simulink library "Lib_Turbo_TurbinePSI_TMATS_org"  (Simulink 10.0)
settings: Solver=ode45  StartTime=0.0  StopTime=10.0  RelTol=1e-3  EnableMultiTasking=on
undefined symbols (not defined in the file): stripchar_TMATS
libraries: Lib_Solve_DataOut_TMATS x1
Description:
  | Thomas Modules
settings Model: Creator=jwchapm2  LastModifiedBy=bhisma

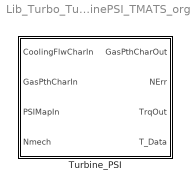
== system Lib_Turbo_TurbinePSI_TMATS_org ==
  Turbine_PSI : Subsystem  mask(T-MATS: Turbine_PSI Library Block){X_T_Map_PRpVec_M=[ 3.000  8.000], Y_T_Map_NcpVec_M=[60 80  110], T_T_Map_PSIArray_M=[0 0; 0 0; 0 0], X_T_Map_PRwVec_M=[ 3.000  8.000], Y_T_Map_NcwVec_M=[60 80  110], T_T_Map_WoWArray_M=[0 0;0 0; 0 0], s_T_hi_M=0.1, s_T_Nc_M=0.0243, s_T_Wc_M=0.4504, s_T_PR_M=0.9736, s_T_Eff_M=0.9984, CFlwEn_M=off, T_CoolFlwPos_M=0, gamma_M=1.4, Rt_M=0.1, iDesign_M=2, NcDes_M=100, EffDes_M=0.9328, PRDes_M=5, NDes_M=10000, FVar_M=strcat('iDes_',stripchar_TMATS(gcb),'.bin')}
      mask prompts: X_T_Map_PRpVec_M "X_T_Map_PRpVec_M - Turbine Map Pressure Ratio Vector (X-axis)(nx1)"; Y_T_Map_NcpVec_M "Y_T_Map_NcpVec_M - Turbine Map Corrected Speed Vector (Y-axis)(mx1)"; T_T_Map_PSIArray_M "T_T_Map_PSIArray_M - Turbine Map PSIMAPI Array (PSIMAPI = f(Nc,PR))(mxn)"; X_T_Map_PRwVec_M "X_T_Map_PRwVec_M - Turbine Map Pressure Ratio Vector (X-axis)(rx1)"; Y_T_Map_NcwVec_M "Y_T_Map_NcwVec_M - Turbine Map Corrected Speed Vector (Y-axis)(qx1)"; T_T_Map_WoWArray_M "T_T_Map_WoWArray_M - Turbine Map Flow Array (WoW=f(Nc,PR))(qxr)"; s_T_hi_M "s_T_hi_M - Corrected Entalpy Constant (T_hi)"; s_T_Nc_M "s_T_Nc_M - Corrected Speed Scalar Constant (T_Nc)"; s_T_Wc_M "s_T_Wc_M - Flow Scalar Constant (T_Wc)"; s_T_PR_M "s_T_PR_M - Pressure Ratio Scalar Constant (T_PR)"; s_T_Eff_M "s_T_Eff_M - Efficiency Scalar Constant (T_Eff)"; CFlwEn_M "CFlwEn_M - Cooling Flow Enable [0-off, 1-on]"; T_CoolFlwPos_M "T_CoolFlwPos_M - Cooling Flow position [0 at inlet,  1 at exit] (cx1)"; iDesign_M "iDesign_M - Design fork (0 - Enable iDes, 1 - Use iDes Scalars, 2 - Use Specified Input Scalars)"; NcDes_M "NcDes_M - Design Corrected Shaft Speed [rpm]"; EffDes_M "EffDes_M - Design Efficiency [frac]"; PRDes_M "PRDes_M - Design Pressure Ratio [frac]"; NDes_M "NDes_M - Design Shaft Speed [rpm]"; FVar_M "FVar_M - File name for iDes Variables"
      mask help: This block simulates the performance of a turbine using basic thermodynamic equations, properties, and table lookups. Turbine_PSI look up tables for this block are based on PSI instead Pressure Ratio as in the Turbine block.
      mask init:
      | if iDesign_M == 1
      |     P = load(FVar_M);
      |     s_T_Nc_M = P(1);
      |     s_T_Wc_M = P(2);
      |     s_T_PR_M = P(3);
      |     s_T_Eff_M = P(4);
      | end
      | 
      | if length(X_T_Map_PRpVec_M) ~= size(T_T_Map_PSIArray_M,2)
      |     warning('number of columns in T_T_Map_PSIArray_M does not match length of X_T_Map_PRVec_M');
      | end
      | if length(X_T_Map_PRwVec_M) ~= size(T_T_Map_WoWArray_M,2)
      |     warning('number of columns in T_T_Map_WoWArray_M does not match length of X_T_Map_PRVec_M');
      | end
      | if length(Y_T_Map_NcpVec_M) ~= size(T_T_Map_PSIArray_M,1)
      |     warning('number of rows in T_T_Map_PSIArray_M does not match length of Y_T_Map_NcVec_M');
      | end
      | if length(Y_T_Map_NcwVec_M) ~= size(T_T_Map_WoWArray_M,1)
      |     warning('number of rows in T_T_Map_WoWArray_M does not match length of Y_T_Map_NcVec_M');
      | end
      mask Help: web(which('Turbo_TMATS_TrbPSI.html'),'-helpbrowser')
      mask Callback CFlwEn_M: MSK_SEC_Enables_TMATS('CFlwEn_M',13,'en')
      mask Callback iDesign_M:
      | MSK_SEC_Enables_Ides_TMATS('iDesign_M',[8 9 10 11],'G1')
      | MSK_SEC_Enables_Ides_TMATS('iDesign_M',[17 18 19 20],'G2')
      | MSK_SEC_Enables_Ides_TMATS('iDesign_M',[21],'G3')

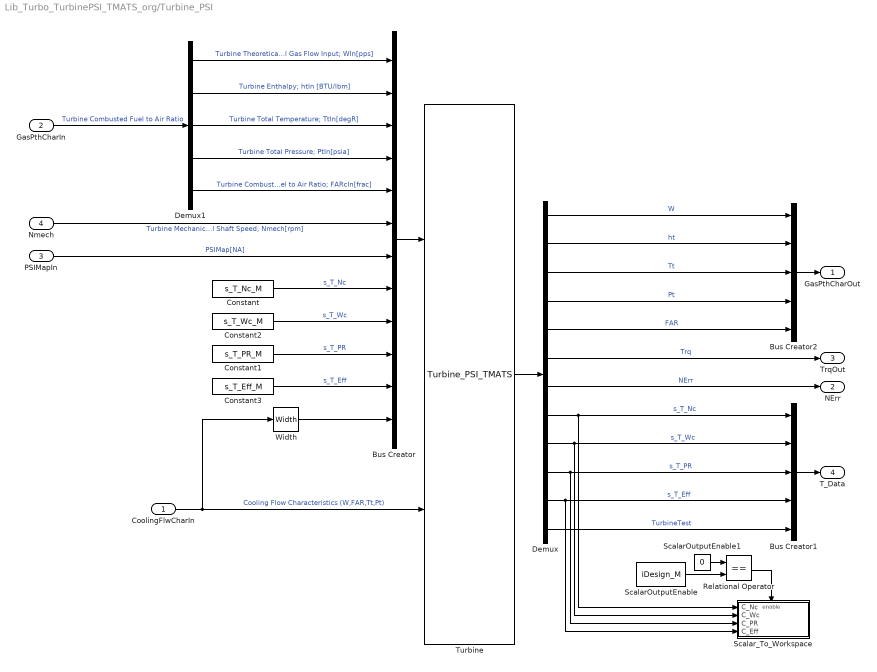
== system Lib_Turbo_TurbinePSI_TMATS_org/Turbine_PSI ==
  CoolingFlwCharIn : Inport
  GasPthCharIn : Inport  Port=2
  PSIMapIn : Inport  Port=3
  Nmech : Inport  Port=4
  Bus Creator : BusCreator  Inputs=12
  Bus Creator1 : BusCreator  Inputs=5
  Bus Creator2 : BusCreator  Inputs=5
  Constant : Constant  Value=s_T_Nc_M
  Constant1 : Constant  Value=s_T_PR_M
  Constant2 : Constant  Value=s_T_Wc_M
  Constant3 : Constant  Value=s_T_Eff_M
  Demux : Demux  Outputs=12
  Demux1 : Demux  Outputs=5
  Relational Operator : RelationalOperator  Operator===  OutDataTypeStr=boolean  RndMeth=Nearest
  ScalarOutputEnable : Constant  Value=iDesign_M
  ScalarOutputEnable1 : Constant  Value=0
  Scalar_To_Workspace : Subsystem
  Turbine : S-Function  FunctionName=Turbine_PSI_TMATS  Parameters=Y_T_Map_NcpVec_M, X_T_Map_PRpVec_M, Y_T_Map_NcwVec_M, X_T_Map_PRwVec_M, T_T_Map_WoWArray_M, T_T_Map_PSIArray_M, T_CoolFlwPos_M, length(T_CoolFlwPos_M), CFlwEn_M, iDesign_M, NcDes_M, EffDes_M, PRDes_M, NDes_M, s_T_hi_M, gamma_M, Rt_M, gcs  SFunctionModules='h2tc_TMATS pt2sc_TMATS sp2tc_TMATS t2hc_TMATS interp2Ac_TMATS functions_TMATS'  SFunctionDeploymentMode=off  EnableBusSupport=off
  Width : Width
  GasPthCharOut : Outport
  NErr : Outport  Port=2
  TrqOut : Outport  Port=3
  T_Data : Outport  Port=4
  wires:
  Demux/11 -> Scalar_To_Workspace/4(C_Eff), Bus Creator1/4  "s_T_Eff"
  Demux/10 -> Scalar_To_Workspace/3(C_PR), Bus Creator1/3  "s_T_PR"
  Demux/9 -> Scalar_To_Workspace/2(C_Wc), Bus Creator1/2  "s_T_Wc"
  Demux/8 -> Scalar_To_Workspace/1(C_Nc), Bus Creator1/1  "s_T_Nc"
  Bus Creator1/1 -> T_Data/1
  Demux1/5 -> Bus Creator/5  "Turbine Combusted Fuel to Air Ratio; FARcIn[frac]"
  CoolingFlwCharIn/1 -> Width/1, Turbine/2  "Cooling Flow Characteristics (W,FAR,Tt,Pt)"
  Demux/7 -> NErr/1  "NErr"
  Demux1/1 -> Bus Creator/1  "Turbine Theoretical Gas Flow Input; WIn[pps]"
  GasPthCharIn/1 -> Demux1/1  "Turbine Combusted Fuel to Air Ratio"
  Bus Creator2/1 -> GasPthCharOut/1
  Demux1/4 -> Bus Creator/4  "Turbine Total Pressure; PtIn[psia]"
  Nmech/1 -> Bus Creator/6  "Turbine Mechanical Shaft Speed; Nmech[rpm]"
  Demux/6 -> TrqOut/1  "Trq"
  Demux/2 -> Bus Creator2/2  "ht"
  Bus Creator/1 -> Turbine/1
  Demux/4 -> Bus Creator2/4  "Pt"
  Demux/3 -> Bus Creator2/3  "Tt"
  Demux/5 -> Bus Creator2/5  "FAR"
  Demux/1 -> Bus Creator2/1  "W"
  Turbine/1 -> Demux/1
  Demux1/3 -> Bus Creator/3  "Turbine Total Temperature; TtIn[degR]"
  Demux1/2 -> Bus Creator/2  "Turbine Enthalpy; htIn [BTU/lbm]"
  PSIMapIn/1 -> Bus Creator/7  "PSIMap[NA]"
  Demux/12 -> Bus Creator1/5  "TurbineTest"
  ScalarOutputEnable/1 -> Relational Operator/2
  ScalarOutputEnable1/1 -> Relational Operator/1
  Relational Operator/1 -> Scalar_To_Workspace/Enable
  Width/1 -> Bus Creator/12
  Constant/1 -> Bus Creator/8  "s_T_Nc"
  Constant1/1 -> Bus Creator/10  "s_T_PR"
  Constant2/1 -> Bus Creator/9  "s_T_Wc"
  Constant3/1 -> Bus Creator/11  "s_T_Eff"

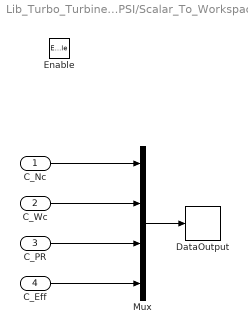
== system Lib_Turbo_TurbinePSI_TMATS_org/Turbine_PSI/Scalar_To_Workspace ==
  C_Nc : Inport
  C_Wc : Inport  Port=2
  C_PR : Inport  Port=3
  C_Eff : Inport  Port=4
  Enable : EnablePort
  DataOutput : Lib_Solve_DataOut_TMATS/DataOutput  FVar_M=FVar_M
  Mux : Mux
  wires:
  C_Eff/1 -> Mux/4
  C_PR/1 -> Mux/3
  C_Wc/1 -> Mux/2
  C_Nc/1 -> Mux/1
  Mux/1 -> DataOutput/1
